simulink model "lmsadlp"  (Simulink 5.0)
settings: Solver=FixedStepDiscrete  SolverMode=SingleTasking  StartTime=0.0  StopTime=999999  RelTol=1e-3  AbsTol=1e-6
libraries: dspsigops x1, dspadpt3 x1, simulink x1, dspsnks4 x1, dspsrcs4 x1
Description:
  | LMS adaptive linear predictor
settings Model: CovMetricSettings=d  Creator=don  LastModifiedBy=mkhan  ExtModeTrigMode=oneshot  ExtModeArmWhenConnect=off  SaveTime=off  SaveOutput=off  LimitDataPoints=off  IntegerOverflowMsg=none  BlockReductionOpt=off  BooleanDataType=off  ZeroCrossControl=UseLocalSettings  TargetHWChar=2  TargetHWWordLengths=8,16,32,32  RTWMathFcnLibMatFile=iso_c_tmw.mat  RTWOptions="-aEnforceIntegerDowncast=1 -aFoldNonRolledExpr=1 -aInlineInvariantSignals=1 -aInlineParameters=0 -aLocalBlockOutputs=1 -aRollThreshold=2 -aRTWVerbose=1 -aForceParamTrailComments=0 -aGenerateComments=1 -aIgnoreCustomStorageClasses=1 -aIncHierarchyInIds=0 -aMaxRTWIdLen=31 -aShowEliminatedStatements=0 -aReadOnly=0 -aTargetFcnLib=\"iso_c_tmw.mat\" -aIncDataTypeInIds=0 -aPrefixModelToSubsysFcnNames=1 -aInlinedPrmAccess=\"Literals\" -aGenerateFullHeader=1 -aIsPILTarget=0 -aGenerateReport=0 -aLogVarNameModifier=\"rt_\" -aExtMode=0 -aExtModeStaticAlloc=0 -aExtModeTesting=0 -aExtModeStaticAllocSize=1000000 -aExtModeTransport=0"

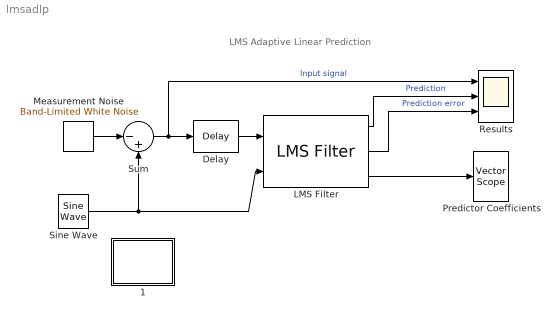
== system lmsadlp ==
  note: LMS Adaptive Linear Prediction
  " 1" : Subsystem
      mask Display: disp('Info')
  Delay : dspsigops/Delay  dly_unit=Samples  delay=1  ic_detail=off  dif_ic_for_ch=off  dif_ic_for_dly=off  ic=0  reset_popup=None
  LMS Filter : dspadpt3/LMS Filter  Algo=Normalized LMS  L=16  stepflag=Dialog  mu=0.5  leakage=1.0  addnparflag=off  ic=0  Adapt=off  resetflag=None  weights=on
  Measurement Noise : simulink/Sources/Band-Limited White Noise  Cov=[0.1]  Ts=1  seed=[23341]
  Predictor Coefficients : dspsnks4/Vector Scope  ScopeProperties=on  Domain=User-defined  HorizSpan=1  DisplayProperties=off  AxisGrid=on  Memory=off  FrameNumber=on  AxisLegend=off  AxisZoom=on  OpenScopeAtSimStart=on  OpenScopeImmediately=off  FigPos=[222 254 343 297]  AxisProperties=off  XUnits=Hertz  XRange=[0...Fs/2]  InheritXIncr=off  XIncr=1  XLabel=Samples  YUnits=dB  YLabel=Amplitude  LineProperties=off
      settings: YMin=-0.2  YMax=0.25
  Results : Scope  NumInputPorts=3
      settings: TimeRange=300  YMin=-2~-2~-0.4  YMax=2~2~1  DataFormat=Array
  Sine Wave : dspsrcs4/Sine Wave  Amplitude=1  Frequency=0.015  Phase=0  SampleMode=Discrete  OutComplex=Real  CompMethod=Trigonometric fcn  TableSize=Speed  SampleTime=1  SamplesPerFrame=1  dataType=double  wordLen=16  udDataType=sfix(16)  fracBitsMode=Best precision  numFracBits=14  ResetState=Restart at time zero
  Sum : Sum  Inputs=|-+  SaturateOnIntegerOverflow=on  InputSameDT=on
  wires:
  Sum/1 -> Results/1, Delay/1  "Input signal"
  LMS Filter/3 -> Predictor Coefficients/1
  Delay/1 -> LMS Filter/1
  Sine Wave/1 -> Sum/2, LMS Filter/2
  Measurement Noise/1 -> Sum/1
  LMS Filter/2 -> Results/3  "Prediction error"
  LMS Filter/1 -> Results/2  "Prediction"

== system lmsadlp/ 1 ==
  note: Adaptive One-Step Linear Prediction
      |
      | This demonstrates the ability of the LMS Adaptive FIR
      | algorithm to adaptively compute the linear prediction
      | coefficients for a noisy input signal.
      |
      | For more information on LMS filtering, see
      | S. Haykin, "Adaptive Filter Theory",
      | 3rd Ed., Prentice Hall, 1996.
